simulink model "kalman"  (R2020b)
settings: Solver=VariableStepAuto  StartTime=0.0  StopTime=10.0  RelTol=1e-3
values from neighbouring files (symbols this model uses):
  C = [1 0]    [kalman_script.m]
  G = [h^2/2; h]    [kalman_script.m]
  Gamma = [h^2/2; h]    [kalman_script.m]
  h = 1    [kalman_script.m]
  Phi = [1 h; 0 1]    [kalman_script.m]
  Q = .001    (= 0.001)    [kalman_script.m]
  R = .001    (= 0.001)    [kalman_script.m]
  x10 = 0    [kalman_script.m]
  x20 = 10    [kalman_script.m]
undefined symbols (not defined in the file or in its folder): Flqr
settings Model: Creator=lucas  LastModifiedBy=lucas

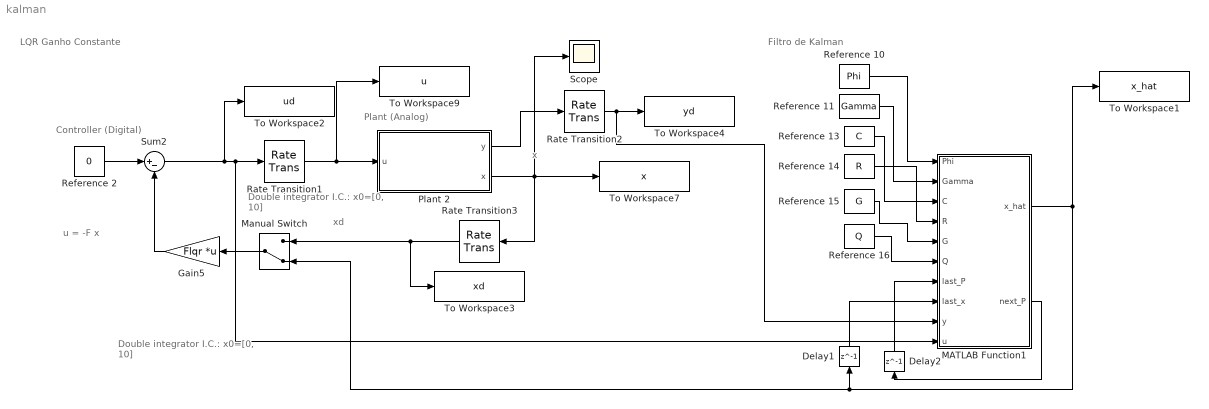
== system kalman ==
  note: Filtro de Kalman
  note: Plant (Analog)
  note: Double integrator
      | I.C.: x0=[0, 10]
  note: x
  note: Controller (Digital)
  note: Double integrator
      | I.C.: x0=[0, 10]
  note: u = -F x
  note: xd
  note: LQR Ganho Constante
  Delay1 : Delay  DelayLength=1  InitialCondition=0  SampleTime=h
  Delay2 : Delay  DelayLength=1  InitialCondition=[1 0;0 1]  SampleTime=h
  Gain5 : Gain  Gain=Flqr  Multiplication=Matrix(K*u)
  MATLAB Function1 : MATLAB Function  TreatAsAtomicUnit=on
  Manual Switch : ManualSwitch  CurrentSetting=0
  Plant 2 : Subsystem
      mask Display:
      | text(.5,.6,'dx/dt = Ax + Bu','horizontalAlignment', 'center','verticalAlignment', 'middle','texmode','on')
      | text(.5,.4,'y = Cx + Du','horizontalAlignment', 'center','verticalAlignment', 'middle','texmode','on')
      | port_label('input',1,'u')
      | port_label('output',1,'y')
      | port_label('output',2,'x')
  Rate Transition1 : RateTransition  Integrity=off  OutPortSampleTime=h_plant
  Rate Transition2 : RateTransition  Integrity=off  OutPortSampleTime=h
  Rate Transition3 : RateTransition  Integrity=off  OutPortSampleTime=h
  Reference 10 : Constant  Value=Phi  VectorParams1D=off  SampleTime=h
  Reference 11 : Constant  Value=Gamma  VectorParams1D=off  SampleTime=h
  Reference 13 : Constant  Value=C  VectorParams1D=off  SampleTime=h
  Reference 14 : Constant  Value=R  VectorParams1D=off  SampleTime=h
  Reference 15 : Constant  Value=G  VectorParams1D=off  SampleTime=h
  Reference 16 : Constant  Value=Q  VectorParams1D=off  SampleTime=h
  Reference 2 : Constant  Value=0  SampleTime=h
  Scope : Scope
  Sum2 : Sum  Inputs=|+-
  To Workspace1 : ToWorkspace  VariableName=x_hat  SaveFormat=Timeseries  SampleTime=-1
  To Workspace2 : ToWorkspace  VariableName=ud  SaveFormat=Timeseries  SampleTime=-1
  To Workspace3 : ToWorkspace  VariableName=xd  SaveFormat=Timeseries  SampleTime=-1
  To Workspace4 : ToWorkspace  VariableName=yd  SaveFormat=Timeseries  SampleTime=-1
  To Workspace7 : ToWorkspace  VariableName=x  SaveFormat=Timeseries  SampleTime=-1
  To Workspace9 : ToWorkspace  VariableName=u  SaveFormat=Timeseries  SampleTime=-1
  wires:
  Plant 2/2(x) -> Rate Transition3/1, To Workspace7/1, Scope/1
  Rate Transition1/1 -> Plant 2/1(u), To Workspace9/1
  Gain5/1 -> Sum2/2
  Reference 2/1 -> Sum2/1
  Rate Transition3/1 -> To Workspace3/1, Manual Switch/1
  Reference 14/1 -> MATLAB Function1/4(R)
  Delay2/1 -> MATLAB Function1/7(last_P)
  Reference 15/1 -> MATLAB Function1/5(G)
  Delay1/1 -> MATLAB Function1/8(last_x)
  Reference 11/1 -> MATLAB Function1/2(Gamma)
  Reference 13/1 -> MATLAB Function1/3(C)
  Reference 16/1 -> MATLAB Function1/6(Q)
  MATLAB Function1/2(next_P) -> Delay2/1
  Sum2/1 -> To Workspace2/1, Rate Transition1/1, MATLAB Function1/10(u)
  Reference 10/1 -> MATLAB Function1/1(Phi)
  Plant 2/1(y) -> Rate Transition2/1
  Manual Switch/1 -> Gain5/1
  MATLAB Function1/1(x_hat) -> Delay1/1, Manual Switch/2, To Workspace1/1
  Rate Transition2/1 -> MATLAB Function1/9(y), To Workspace4/1

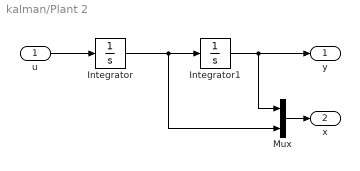
== system kalman/Plant 2 ==
  u : Inport
  Integrator : Integrator  InitialCondition=x20
  Integrator1 : Integrator  InitialCondition=x10
  Mux : Mux  Inputs=2
  y : Outport
  x : Outport  Port=2
  wires:
  Integrator/1 -> Mux/2, Integrator1/1
  Integrator1/1 -> Mux/1, y/1
  u/1 -> Integrator/1
  Mux/1 -> x/1

== matlab function kalman/MATLAB Function1 ==
  data: Phi input size=[2 2]; Gamma input size=[2 1]; C input size=[1 2]; R input size=1; G input size=[2 1]; Q input size=1; last_P input size=[2 2]; x_hat output size=[2 1]; last_x input size=[2 1]; y input size=1; u input size=1; next_P output size=[2 2]
    function [x_hat, next_P] = fcn(Phi, Gamma, C, R, G, Q, last_P, last_x, y, u)

P = inv(last_P) + C'*inv(R)*C;
P = inv(P);
next_P = Phi*P*Phi' + G*Q*G';
L = P*C'*inv(R);
x = last_x + L*(y - C*last_x);
x_hat = Phi*x + Gamma*u;
